simulink model "chap1_19"  (R2016a)
settings: Solver=ode4  StartTime=0.0  StopTime=1  FixedStep=ts  RelTol=1e-3
values from neighbouring files (symbols this model uses):
  ki = 0.80    (= 0.8)    [Discrete_Kalman_filter_for_PID_control.m]    (also in Integration_Separation_PID_Controller.m = 0.005; PID_CTR_Z_transform.m = 0.1; PID_Controller_for_square_tracking_with_filtered_signal.m = 0.002; PID_Controller_with _intergration_sturation.m = 9)
  kp = 8.0    (= 8)    [Discrete_Kalman_filter_for_PID_control.m]    (also in Integration_Separation_PID_Controller.m = 0.8; PID_CTR_Z_transform.m; PID_Controller_for_square_tracking_with_filtered_signal.m = 0.8; PID_Controller_with _intergration_sturation.m = 0.85)
  ts = 0.5    [Delay_Control_with_Dalin_Algorithm.m]    (also in Discrete_Kalman_filter_for_PID_control.m = 0.001; Filter_with_tracker_and_differentiation.m = 0.001; Integration_Separation_PID_Controller.m = 20; Kalman_filter.m = 0.001)
undefined symbols (not defined in the file or in its folder): den, denQ, DiscIntNeverNeededParam, num, numQ
settings Model: Creator=admin  LastModifiedBy=admin

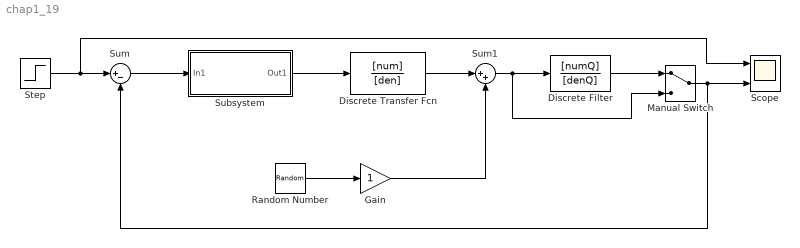
== system chap1_19 ==
  Discrete Transfer Fcn : DiscreteTransferFcn  Numerator=[num]  Denominator=[den]  SampleTime=ts
  Discrete Filter : DiscreteFilter  Numerator=[numQ]  Denominator=[denQ]  SampleTime=ts
  Gain : Gain
  Manual Switch : ManualSwitch
  Random Number : RandomNumber  SampleTime=ts
  Scope : Scope  NumInputPorts=2
  Step : Step  Time=0  After=20  SampleTime=ts
  Subsystem : Subsystem
  Sum : Sum  Inputs=|+-
  Sum1 : Sum  Inputs=|++
  wires:
  Sum/1 -> Subsystem/1(In1)
  Step/1 -> Scope/1, Sum/1
  Subsystem/1(Out1) -> Discrete Transfer Fcn/1
  Discrete Transfer Fcn/1 -> Sum1/1
  Random Number/1 -> Gain/1
  Gain/1 -> Sum1/2
  Sum1/1 -> Manual Switch/2, Discrete Filter/1
  Discrete Filter/1 -> Manual Switch/1
  Manual Switch/1 -> Scope/2, Sum/2

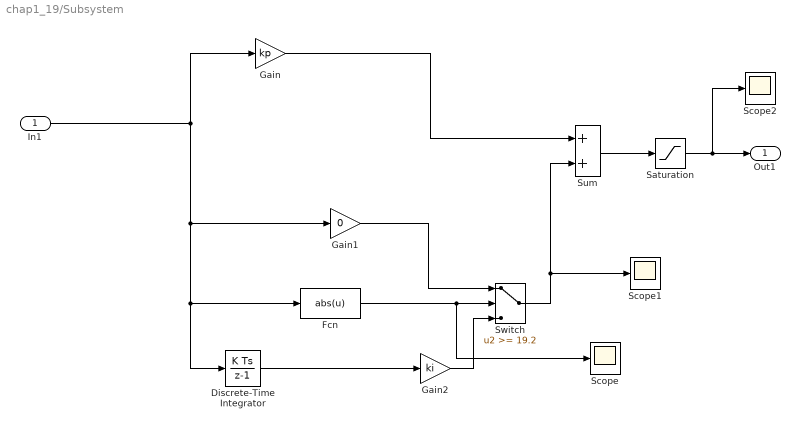
== system chap1_19/Subsystem ==
  In1 : Inport
  Discrete-Time Integrator : DiscreteIntegrator  InitialConditionSetting=State (most efficient)  SampleTime=ts  ICPrevOutput=DiscIntNeverNeededParam  ICPrevScaledInput=DiscIntNeverNeededParam
  Fcn : Fcn  Expr=abs(u)
  Gain : Gain  Gain=kp
  Gain1 : Gain  Gain=0
  Gain2 : Gain  Gain=ki
  Saturation : Saturate  UpperLimit=10  LowerLimit=-10
  Scope : Scope
  Scope1 : Scope
  Scope2 : Scope
  Sum : Sum
  Switch : Switch  Threshold=19.2
  Out1 : Outport
  wires:
  Discrete-Time Integrator/1 -> Gain2/1
  In1/1 -> Discrete-Time Integrator/1, Fcn/1, Gain1/1, Gain/1
  Fcn/1 -> Switch/2, Scope/1
  Gain2/1 -> Switch/3
  Gain1/1 -> Switch/1
  Gain/1 -> Sum/1
  Switch/1 -> Scope1/1, Sum/2
  Sum/1 -> Saturation/1
  Saturation/1 -> Scope2/1, Out1/1
